simulink subsystem "filter_2s3o"  (R2021b)
settings: Solver=VariableStepAuto  StartTime=0.0  StopTime=10.0  RelTol=1e-3
settings Model: Creator=torha  LastModifiedBy=torha

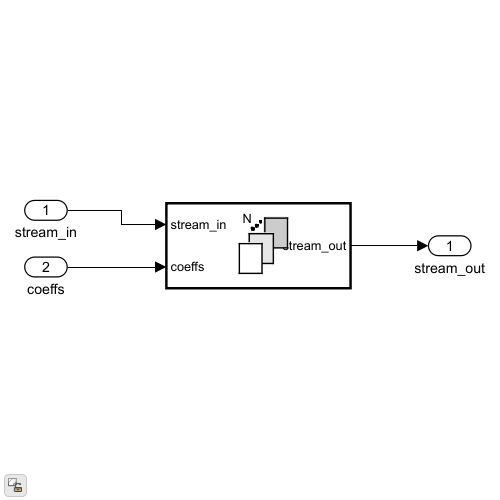
[thumbnail: Simulink's stored preview of the top-level diagram]
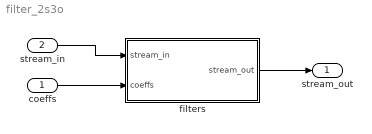
== system filter_2s3o ==
  coeffs : Inport
  stream_in : Inport  Port=2
  filters : Subsystem
  stream_out : Outport
  wires:
  filters/1(stream_out) -> stream_out/1
  coeffs/1 -> filters/2(coeffs)
  stream_in/1 -> filters/1(stream_in)

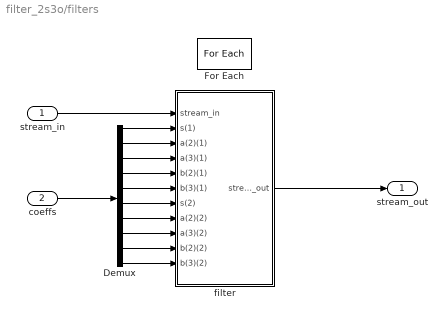
== system filter_2s3o/filters ==
  stream_in : Inport  Partition=on  PartitionDimension=2  PartitionWidth=1  PartitionOffset=0
  coeffs : Inport  Port=2
  Demux : Demux  Outputs=10
  For Each : ForEach  DisableCoverage=on
  filter : Subsystem
  stream_out : Outport  ConcatenationDimension=1
  wires:
  Demux/10 -> filter/11(b(3)(2))
  Demux/9 -> filter/10(b(2)(2))
  Demux/8 -> filter/9(a(3)(2))
  Demux/7 -> filter/8(a(2)(2))
  Demux/6 -> filter/7(s(2))
  Demux/5 -> filter/6(b(3)(1))
  Demux/4 -> filter/5(b(2)(1))
  Demux/3 -> filter/4(a(3)(1))
  Demux/2 -> filter/3(a(2)(1))
  Demux/1 -> filter/2(s(1))
  stream_in/1 -> filter/1(stream_in)
  coeffs/1 -> Demux/1
  filter/1(stream_out) -> stream_out/1

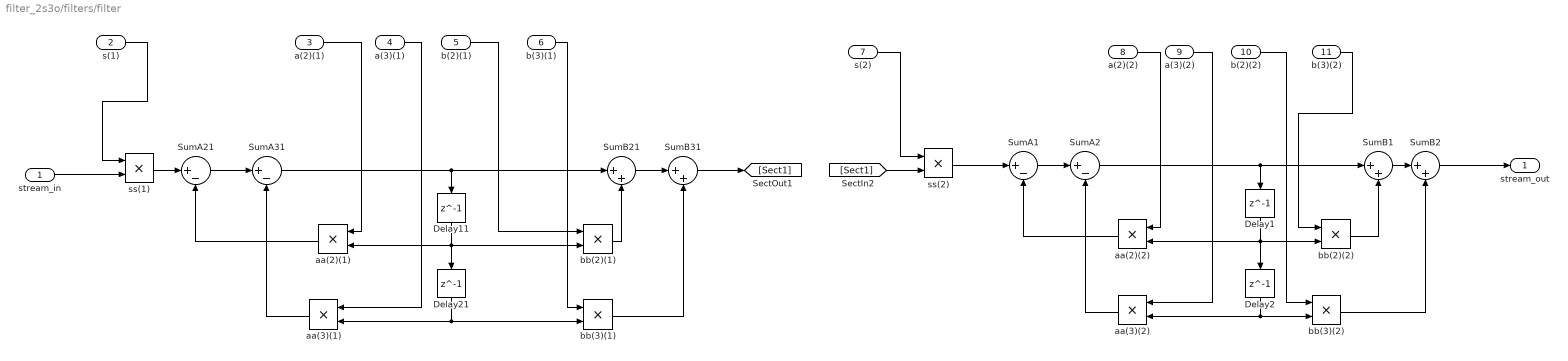
== system filter_2s3o/filters/filter ==
  stream_in : Inport
  s(1) : Inport  Port=2
  a(2)(1) : Inport  Port=3
  a(3)(1) : Inport  Port=4
  b(2)(1) : Inport  Port=5
  b(3)(1) : Inport  Port=6
  s(2) : Inport  Port=7
  a(2)(2) : Inport  Port=8
  a(3)(2) : Inport  Port=9
  b(2)(2) : Inport  Port=10
  b(3)(2) : Inport  Port=11
  Delay{1..2,11,21} (4 alike) : Delay  DelayLength=1  InitialCondition=0
  SumA{1..2,21,31} (4 alike) : Sum  Inputs=|+-  RndMeth=Nearest  SaturateOnIntegerOverflow=on  OutDataTypeStr=Inherit: Same as first input
  SumB{1..2,21,31} (4 alike) : Sum  Inputs=|++  RndMeth=Nearest  SaturateOnIntegerOverflow=on  OutDataTypeStr=Inherit: Same as first input
  aa(2)(1) : Product
  aa(2)(2) : Product
  aa(3)(1) : Product
  aa(3)(2) : Product
  bb(2)(1) : Product
  bb(2)(2) : Product
  bb(3)(1) : Product
  bb(3)(2) : Product
  ss(1) : Product
  ss(2) : Product
  stream_out : Outport
  wires:
  b(2)(2)/1 -> bb(3)(2)/1
  SumB2/1 -> stream_out/1
  b(3)(2)/1 -> bb(2)(2)/1
  a(2)(2)/1 -> aa(2)(2)/1
  b(2)(1)/1 -> bb(2)(1)/1
  bb(2)(2)/1 -> SumB1/2
  aa(2)(1)/1 -> SumA21/2
  SumB31/1 -> [Sect1]
  SumB21/1 -> SumB31/1
  a(3)(1)/1 -> aa(3)(1)/1
  a(2)(1)/1 -> aa(2)(1)/1
  SumA1/1 -> SumA2/1
  SumA21/1 -> SumA31/1
  SumB1/1 -> SumB2/1
  s(2)/1 -> ss(2)/1
  ss(1)/1 -> SumA21/1
  bb(2)(1)/1 -> SumB21/2
  b(3)(1)/1 -> bb(3)(1)/1
  aa(3)(1)/1 -> SumA31/2
  aa(3)(2)/1 -> SumA2/2
  bb(3)(2)/1 -> SumB2/2
  a(3)(2)/1 -> aa(3)(2)/1
  Delay1/1 -> bb(2)(2)/2, Delay2/1, aa(2)(2)/2
  stream_in/1 -> ss(1)/2
  ss(2)/1 -> SumA1/1
  [Sect1] -> ss(2)/2
  Delay11/1 -> Delay21/1, bb(2)(1)/2, aa(2)(1)/2
  SumA2/1 -> SumB1/1, Delay1/1
  Delay21/1 -> bb(3)(1)/2, aa(3)(1)/2
  bb(3)(1)/1 -> SumB31/2
  SumA31/1 -> SumB21/1, Delay11/1
  s(1)/1 -> ss(1)/1
  aa(2)(2)/1 -> SumA1/2
  Delay2/1 -> bb(3)(2)/2, aa(3)(2)/2
